simulink model "omarssoluutionslx"  (R2016a)
settings: Solver=VariableStepAuto  StartTime=0.0  StopTime=10.0  RelTol=1e-3
values from neighbouring files (symbols this model uses):
  A = [0 1 0 0; -k1/J1 -c1/J1 k1/J1 0;0 0 0 1; k1/J2 0 (-k1-k2)/J2 -c2/J2;]    [Controllable.m]    (also in ControllableV1.m = [0 1 0 0; ControllableV2.m = [0 1 0 0)
  B = [0; 1/J1; 0; 0;]    [Controllable.m]    (also in ControllableV1.m; ControllableV2.m)
  C = eye(4)    [Controllable.m]    (also in ControllableV1.m; ControllableV2.m)
  D = [0;0;0;0;]    [Controllable.m]    (also in ControllableV1.m; ControllableV2.m)
libraries: simulink x1
settings Model: Creator=ramik  LastModifiedBy=ramik

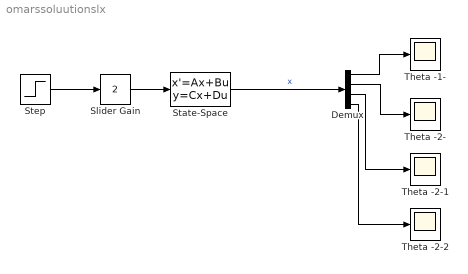
== system omarssoluutionslx ==
  Demux : Demux
  Slider Gain : simulink/Math Operations/Slider Gain  low=0  gain=2  high=2
  State-Space : StateSpace  A=A  B=B  C=C  D=D  X0=0
  Step : Step  SampleTime=0
  Theta -1- : Scope
  Theta -2- : Scope
  Theta -2-1 : Scope
  Theta -2-2 : Scope
  wires:
  Step/1 -> Slider Gain/1
  Slider Gain/1 -> State-Space/1
  Demux/1 -> Theta -1-/1
  Demux/2 -> Theta -2-/1
  State-Space/1 -> Demux/1  "x"
  Demux/3 -> Theta -2-1/1
  Demux/4 -> Theta -2-2/1
